simulink model "mariomodel"  (R2013a)
settings: Solver=ode3  SolverMode=SingleTasking  StartTime=0.0  StopTime=10.0  RelTol=1e-3
PreLoadFcn:
  | Ts = 0.1;
libraries: legonxtlib x4
settings Model: ExtModeTrigDuration=2  Creator=scastro  LastModifiedBy=scastro
settings OptimizationCC: OptimizeModelRefInitCode=on  LifeSpan=1
settings DebuggingCC: SolverPrmCheckMsg=none  StrictBusMsg=Warning
settings HardwareCC: ProdLargestAtomicInteger=Long  ProdLargestAtomicFloat=Float  ProdEndianess=LittleEndian  ProdHWDeviceType=ARM Compatible->ARM 7
settings RTWCC: SystemTargetFile=realtime.tlc  GenerateMakefile=off  TemplateMakefile=realtime.tmf  Description=Run on Target Hardware  RTWVerbose=off  ProcessScript=realtime_make_rtw_hook
settings STFCustomTargetCC: TargetLibSuffix=.a  GenerateSampleERTMain=on  ERTCustomFileBanners=on  SupportNonInlinedSFcns=off  SupportVariableSizeSignals=on  MATLABClassNameForMDSCustomization=Simulink.SoftwareTarget.ERTCustomization  SystemTargetFile=realtime.tlc
settings ERTTargetCC: ParMdlRefBuildCompliant=off  CompOptLevelCompliant=off  ConcurrentExecutionCompliant=off  CombineOutputUpdateFcns=off  ERTFirstTimeCompliant=off  SupportContinuousTime=on  SupportVariableSizeSignals=on  ModelStepFunctionPrototypeControlCompliant=off  CPPClassGenCompliant=off  ExtModeTransport=1  ExtModeMexFile=ext_serial_win32_comm_no_acks_rtt_byteswap  ExtModeMexArgs=0 1 9600  ERTSrcFileBannerTemplate=realtime_code_template.cgt  ERTHdrFileBannerTemplate=realtime_code_template.cgt  ERTDataSrcFileTemplate=realtime_code_template.cgt  ERTDataHdrFileTemplate=realtime_code_template.cgt  ERTCustomFileTemplate=realtime_file_process.tlc

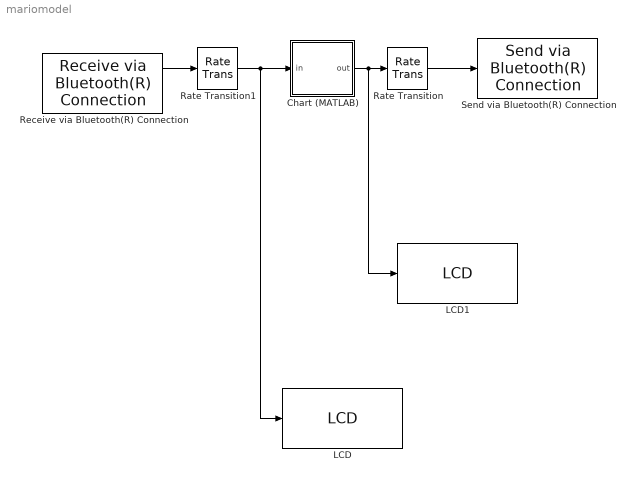
== system mariomodel ==
  Chart (MATLAB) : Stateflow chart  TreatAsAtomicUnit=on
  LCD : legonxtlib/LCD  slcdStr=In  slcdLine=1  slcdFormat=Decimal
  LCD1 : legonxtlib/LCD  slcdStr=Out  slcdLine=2  slcdFormat=Decimal
  Rate Transition : RateTransition  OutPortSampleTime=Ts
  Rate Transition1 : RateTransition  OutPortSampleTime=0.004
  Receive via Bluetooth(R) Connection : legonxtlib/Receive via Bluetooth(R) Connection  mailbox=3  dataType=uint8  dataSize=1  sampleTime=Ts
  Send via Bluetooth(R) Connection : legonxtlib/Send via Bluetooth(R) Connection  mailbox=4
  wires:
  Receive via Bluetooth(R) Connection/1 -> Rate Transition1/1
  Rate Transition/1 -> Send via Bluetooth(R) Connection/1
  Chart (MATLAB)/1(out) -> LCD1/1, Rate Transition/1
  Rate Transition1/1 -> Chart (MATLAB)/1(in), LCD/1

== stateflow chart mariomodel/Chart (MATLAB) ==
  state s8
  state Wait
  state s7
    en:out=uint8(15);
  state s1
    en:out=uint8(11);
  state s6
    en:out=uint8(14);
  state s2
    en:out=uint8(12);
  state s5
  state s3
  state s4
    en:out=uint8(16);
  (default) -> Wait
  s7 -> s8 : [isequal(in,uint8(21))]
  Wait -> s1 : after(10,sec)
  s6 -> s7 : after(5,sec)
  s1 -> s2 : after(5,sec)
  s5 -> s6 : after(5,sec)
  s2 -> s3 : [isequal(in,uint8(20))]
  s4 -> s5 : [isequal(in,uint8(21))]
  s3 -> s4 : after(5,sec)
  data: in input; out output
